simulink subsystem "bare_recv_QPSK"  (R2024b)
settings: Solver=VariableStepAuto  StartTime=0.0  StopTime=10.0  RelTol=1e-3
undefined symbols (not defined in the file or in its folder): frameType, Param
libraries: commrfcorlib x2, commsync2 x2, dspstat3 x2, commrflib2 x1, commutil2 x1, commdigbbndpm3 x1, commfilt2 x1
settings Model: Creator=rober  LastModifiedBy=fredr

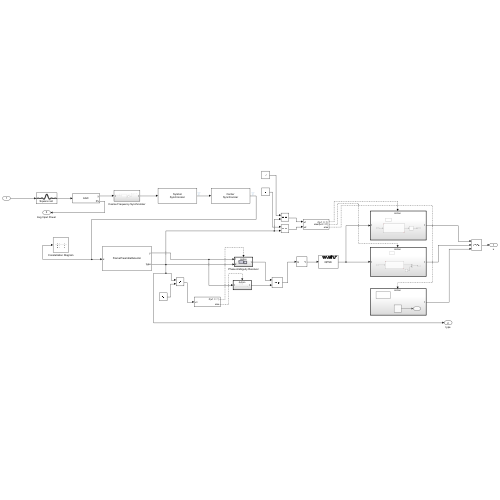
[thumbnail: Simulink's stored preview of the top-level diagram]
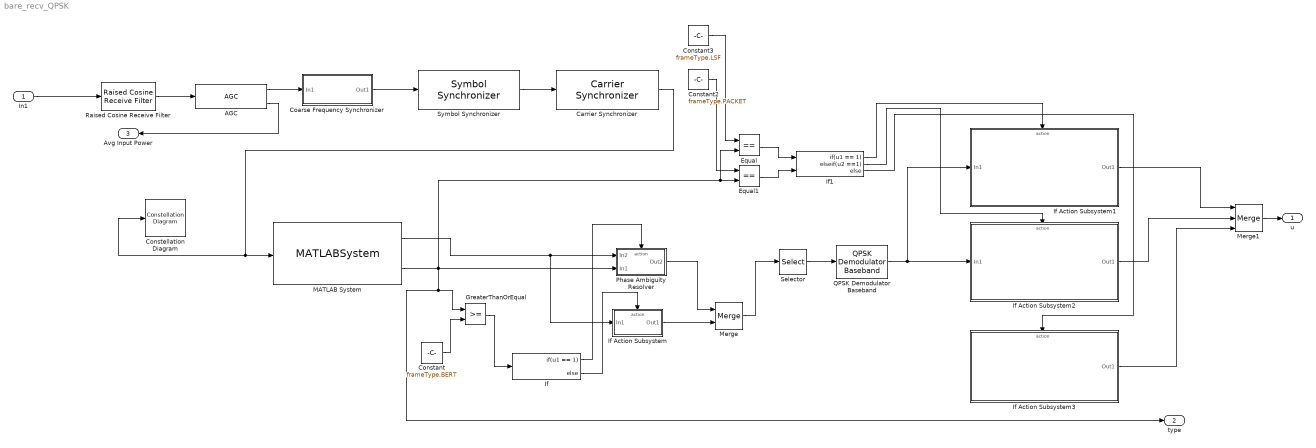
== system bare_recv_QPSK ==
  In1 : Inport  OutDataTypeStr=double
  AGC : commrfcorlib/AGC  LegacyMode=off  DetectorMethod=Rectifier  LoopMethod=Linear  UpdatePeriod=100  StepSize=0.1  AdaptationStepSize=0.01  DesiredOutputPower=2  AveragingLength=Param.AveragingLength*2  MaximumGain=30  MaxPowerGain=20  GainOutputPort=off  InputPowerOutputPort=on  SimulateUsing=Code generation
  Carrier Synchronizer : commsync2/Carrier Synchronizer  Modulation=QPSK  ModulationPhaseOffset=Auto  CustomPhaseOffset=0  SamplesPerSymbol=Param.Interpolation/Param.Decimation  DampingFactor=1  NormalizedLoopBandwidth=0.01  EstimatedPhaseErrorOutputPort=off  SimulateUsing=Code generation
  Coarse Frequency Synchronizer : Subsystem
  Constant : Constant  Value=frameType.BERT
  Constant2 : Constant  Value=frameType.PACKET
  Constant3 : Constant  Value=frameType.LSF
  Constellation Diagram : ConstellationDiagram  WindowPosition=[382.000000,84.000000,600.000000,600.000000,]  Visible=on  ScopeFrameLocation=window  DefaultConfigurationName=comm.scopes.ConstellationDiagramBlockCfg
  Equal : RelationalOperator  Operator===  OutDataTypeStr=boolean  RndMeth=Simplest  InputSameDT=off
  Equal1 : RelationalOperator  Operator===  OutDataTypeStr=boolean  RndMeth=Simplest  InputSameDT=off
  GreaterThanOrEqual : RelationalOperator  OutDataTypeStr=boolean  RndMeth=Simplest  InputSameDT=off
  If : If  IfExpression=u1 == 1
  If Action Subsystem : Subsystem  TreatAsAtomicUnit=on
  If Action Subsystem1 : Subsystem  TreatAsAtomicUnit=on
  If Action Subsystem2 : Subsystem  TreatAsAtomicUnit=on
  If Action Subsystem3 : Subsystem  TreatAsAtomicUnit=on
  If1 : If  NumInputs=2  IfExpression=u1 == 1  ElseIfExpressions=u2 ==1
  MATLAB System : MATLABSystem  System=FramePreambleDetector  EOTPattern=Param.EOT.EoTSymbols  PreamblePattern=Param.Preambles.LSFSymbol  LSFSyncBurst=Param.SyncBurst.LSFSymbol  BERTSyncBurst=Param.SyncBurst.BERTSymbol  StreamSyncBurst=Param.SyncBurst.StreamSymbol  PacketSyncBurst=Param.SyncBurst.PacketSymbol  FrameLength=192  ThresholdMetric=10  SimulateUsing=Interpreted execution
      mask Type: FramePreambleDetector
      mask Display:
      | disp('FramePreambleDetector');
      | port_label('input',1,'x');
      | port_label('output',1,'y');
      | port_label('output',2,'type');
  Merge : Merge
  Merge1 : Merge  Inputs=3
  Phase Ambiguity Resolver : Subsystem  TreatAsAtomicUnit=on
  QPSK Demodulator Baseband : commdigbbndpm3/QPSK Demodulator Baseband  OutType=Bit  DecType=Hard decision  VarSource=Dialog  Variance=1  Dec=Binary  Ph=pi/4  outDtype1=Inherit via internal rule  outDtype2=Inherit via internal rule  derotateFactorWordLen=16  derotateFactorDataTypeStr=Inherit: Same word length as input  derotateFactorLastDataTypeStr=Inherit: Same word length as input
      settings: LibrarySourceBlock=|
      | commhdldigbbndpm/QPSK
      | Demodulator
      | Baseband
  Raised Cosine Receive Filter : commfilt2/Raised Cosine Receive Filter  filtType=Square root  R=Param.RolloffFactor  filtSpan=Param.RaisedCosineFilterSpan  N=Param.Interpolation  downFactor=Param.Decimation  downOffset=0  filterGain=1  InputProcessing=Columns as channels (frame based)  RateOptions=Enforce single-rate processing  framing=Mute  checkCoeff=off  variableName=rcRxFilt  currentFiltSpan=10  D=5  inputOffset=0  sampMode=Mute  saveAsFlag=0  rateMode=Downsampling  checkGain=Normalized  launchFVT=on  roundingMode=Floor  overflowMode=off  coeffDataTypeStr=Inherit: Same word length as input  coeffMin=[]  coeffMax=[]  coeffLastDataTypeStr=Inherit: Same word length as input  accumDataTypeStr=Inherit: Same as product output  accumLastDataTypeStr=Inherit: Same as product output  outputDataTypeStr=Inherit: Same as accumulator  outputMin=[]  outputMax=[]  outputLastDataTypeStr=Inherit: Same as accumulator
  Selector : Selector  IndexOptions=Index vector (dialog)  Indices=[9:192]  OutputSizes=1
  Symbol Synchronizer : commsync2/Symbol Synchronizer  Modulation=PAM/PSK/QAM  TimingErrorDetector=Gardner (non-data-aided)  SamplesPerSymbol=Param.Interpolation/Param.Decimation  DampingFactor=1  NormalizedLoopBandwidth=0.01  DetectorGain=Param.TimingErrorDetectorGain  TimingErrorOutputPort=off  SimulateUsing=Code generation
  u : Outport
  type : Outport  Port=2
  Avg Input Power : Outport  Port=3
  wires:
  MATLAB System/1 -> Phase Ambiguity Resolver/1(In2), If Action Subsystem/1(In1)
  Coarse Frequency Synchronizer/1(Out1) -> Symbol Synchronizer/1
  Symbol Synchronizer/1 -> Carrier Synchronizer/1
  AGC/1 -> Coarse Frequency Synchronizer/1(In1)
  Raised Cosine Receive Filter/1 -> AGC/1
  In1/1 -> Raised Cosine Receive Filter/1
  Phase Ambiguity Resolver/1(Out2) -> Merge/1
  If/1 -> Phase Ambiguity Resolver/Action
  If/2 -> If Action Subsystem/Action
  If Action Subsystem/1(Out1) -> Merge/2
  If1/1 -> If Action Subsystem1/Action
  If1/2 -> If Action Subsystem2/Action
  If1/3 -> If Action Subsystem3/Action
  Merge1/1 -> u/1
  QPSK Demodulator Baseband/1 -> If Action Subsystem2/1(In1), If Action Subsystem1/1(In1)
  Selector/1 -> QPSK Demodulator Baseband/1
  MATLAB System/2 -> Phase Ambiguity Resolver/2(In1), type/1, GreaterThanOrEqual/1, Equal1/2, Equal/2
  Carrier Synchronizer/1 -> MATLAB System/1, Constellation Diagram/1
  If Action Subsystem1/1(Out1) -> Merge1/1
  If Action Subsystem3/1(Out1) -> Merge1/3
  Constant/1 -> GreaterThanOrEqual/2
  GreaterThanOrEqual/1 -> If/1
  Constant2/1 -> Equal1/1
  Constant3/1 -> Equal/1
  Equal/1 -> If1/1
  Equal1/1 -> If1/2
  If Action Subsystem2/1(Out1) -> Merge1/2
  Merge/1 -> Selector/1
  AGC/2 -> Avg Input Power/1

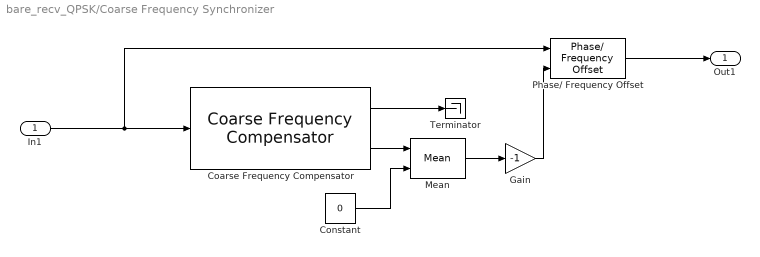
== system bare_recv_QPSK/Coarse Frequency Synchronizer ==
  In1 : Inport
  Coarse Frequency Compensator : commrfcorlib/Coarse Frequency Compensator  Modulation=QPSK  Algorithm=FFT-based  FrequencyResolution=1000  MaximumFrequencyOffset=Param.MaximumFrequencyOffset  SamplesPerSymbol=4  EstimatedFreqOffsetPort=on  SimulateUsing=Code generation
  Constant : Constant  Value=0
  Gain : Gain  Gain=-1
  Mean : dspstat3/Mean  run=on  InputProcessing=Columns as channels (frame based)  reset_popup=Rising edge  directionMode=Each column  dimension=1  roiEnable=off  roiType=Rectangles  roiPortion=Entire ROI  roiOutput=Individual statistics for each ROI  roiFlag=off  roundingMode=Floor  overflowMode=off  outputDataTypeStr=Inherit: Same as accumulator  outputMin=[]  outputMax=[]  outputLastDataTypeStr=Inherit: Same as accumulator
  Phase/ Frequency Offset : commrflib2/Phase// Frequency Offset  phaseOffset=0  freqPort=on  freqOffset=0
  Terminator : Terminator
  Out1 : Outport
  wires:
  In1/1 -> Phase/ Frequency Offset/1, Coarse Frequency Compensator/1
  Mean/1 -> Gain/1
  Coarse Frequency Compensator/2 -> Mean/1
  Gain/1 -> Phase/ Frequency Offset/2
  Phase/ Frequency Offset/1 -> Out1/1
  Coarse Frequency Compensator/1 -> Terminator/1
  Constant/1 -> Mean/2

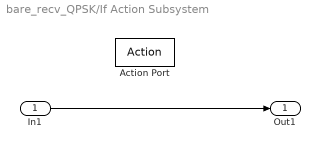
== system bare_recv_QPSK/If Action Subsystem ==
  In1 : Inport
  Action Port : ActionPort
  Out1 : Outport
  wires:
  In1/1 -> Out1/1

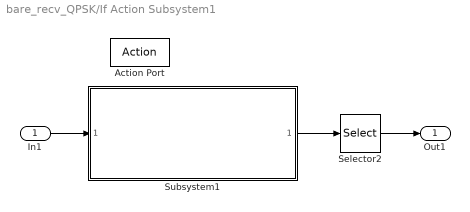
== system bare_recv_QPSK/If Action Subsystem1 ==
  In1 : Inport
  Action Port : ActionPort
  Selector2 : Selector  IndexOptions=Index vector (dialog)  Indices=[1:240]  OutputSizes=1
  Subsystem1 : Subsystem  ReferencedSubsystem=ConvolutionalDecodingLSF
  Out1 : Outport
  wires:
  Selector2/1 -> Out1/1
  Subsystem1/1 -> Selector2/1
  In1/1 -> Subsystem1/1

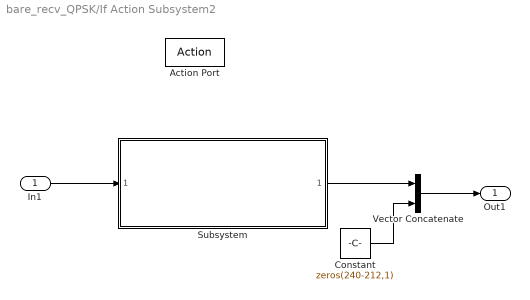
== system bare_recv_QPSK/If Action Subsystem2 ==
  In1 : Inport
  Action Port : ActionPort
  Constant : Constant  Value=zeros(240-212,1)
  Subsystem : Subsystem  ReferencedSubsystem=ConvolutionalDecoding
  Vector Concatenate : Concatenate
  Out1 : Outport
  wires:
  Vector Concatenate/1 -> Out1/1
  Constant/1 -> Vector Concatenate/2
  Subsystem/1 -> Vector Concatenate/1
  In1/1 -> Subsystem/1

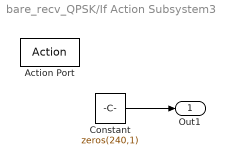
== system bare_recv_QPSK/If Action Subsystem3 ==
  Action Port : ActionPort
  Constant : Constant  Value=zeros(240,1)  VectorParams1D=off
  Out1 : Outport
  wires:
  Constant/1 -> Out1/1

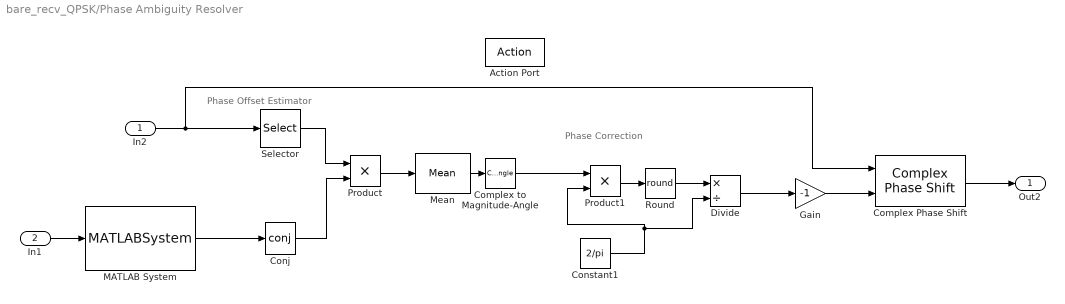
== system bare_recv_QPSK/Phase Ambiguity Resolver ==
  note: Phase Correction
  note: Phase Offset Estimator
  In2 : Inport
  In1 : Inport  Port=2
  Action Port : ActionPort
  Complex Phase Shift : commutil2/Complex Phase Shift
  Complex to Magnitude-Angle : ComplexToMagnitudeAngle  Output=Angle
  Conj : Math  Operator=conj
  Constant1 : Constant  Value=2/pi  VectorParams1D=off
  Divide : Product  Inputs=*/
  Gain : Gain  Gain=-1
  MATLAB System : MATLABSystem  System=SelectHeader  LSFSyncBurst=Param.SyncBurst.LSFSymbol  BERTSyncBurst=Param.SyncBurst.BERTSymbol  StreamSyncBurst=Param.SyncBurst.StreamSymbol  PacketSyncBurst=Param.SyncBurst.PacketSymbol  SimulateUsing=Code generation
      mask Type: SelectHeader
      mask Display:
      | disp('SelectHeader');
      | port_label('input',1,'x');
      | port_label('output',1,'y');
  Mean : dspstat3/Mean  run=off  InputProcessing=Columns as channels (frame based)  reset_popup=None  directionMode=Each column  dimension=1  roiEnable=off  roiType=Rectangles  roiPortion=Entire ROI  roiOutput=Individual statistics for each ROI  roiFlag=off  roundingMode=Floor  overflowMode=off  outputDataTypeStr=Inherit: Same as accumulator  outputMin=[]  outputMax=[]  outputLastDataTypeStr=Inherit: Same as accumulator
  Product : Product
  Product1 : Product
  Round : Rounding  Operator=round
  Selector : Selector  IndexOptions=Index vector (dialog)  Indices=[1:length(Param.SyncBurst.LSF)]  OutputSizes=1
  Out2 : Outport
  wires:
  Product/1 -> Mean/1
  Round/1 -> Divide/1
  Gain/1 -> Complex Phase Shift/2
  In2/1 -> Complex Phase Shift/1, Selector/1
  Divide/1 -> Gain/1
  Mean/1 -> Complex to Magnitude-Angle/1
  Complex Phase Shift/1 -> Out2/1
  Conj/1 -> Product/2
  Selector/1 -> Product/1
  Product1/1 -> Round/1
  Complex to Magnitude-Angle/1 -> Product1/1
  Constant1/1 -> Product1/2, Divide/2
  MATLAB System/1 -> Conj/1
  In1/1 -> MATLAB System/1
